simulink model "Exp5_MODEL_DCDC"  (R2023b)
settings: Solver=ode3  StartTime=0.0  StopTime=Time(end)  FixedStep=1e-6  RelTol=1e-3
undefined symbols (not defined in the file): C, L, LT1D_R_LOAD_1B, LT1D_R_LOAD_2B, R_L, R_lo_C, R_lo_nC_1B, R_lo_nC_2B, U_D, U_out
settings Model: Creator=tunkarlu  LastModifiedBy=tunkarlu

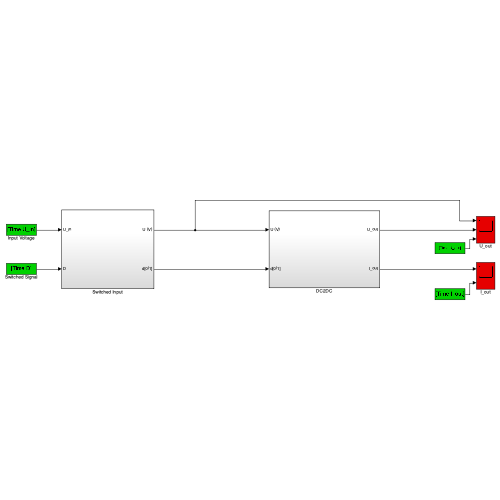
[thumbnail: Simulink's stored preview of the top-level diagram]
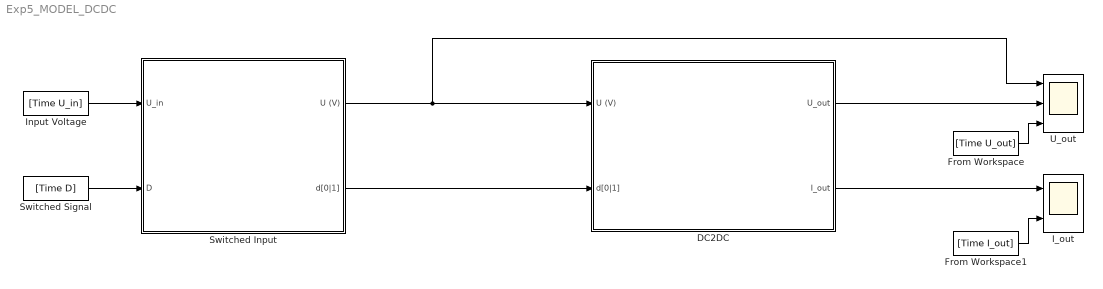
== system Exp5_MODEL_DCDC ==
  DC2DC : Subsystem
  From Workspace : FromWorkspace  VariableName=[Time U_out]
  From Workspace1 : FromWorkspace  VariableName=[Time I_out]
  I_out : Scope  NumInputPorts=2
  Input Voltage : FromWorkspace  VariableName=[Time U_in]
  Switched Input : Subsystem
  Switched Signal : FromWorkspace  VariableName=[Time D]
  U_out : Scope  NumInputPorts=3
  wires:
  Switched Signal/1 -> Switched Input/2(D)
  Input Voltage/1 -> Switched Input/1(U_in)
  From Workspace/1 -> U_out/3
  From Workspace1/1 -> I_out/2
  Switched Input/1(U (V)) -> U_out/1, DC2DC/1(U (V))
  Switched Input/2(d[0|1]) -> DC2DC/2(d[0|1])
  DC2DC/2(I_out) -> I_out/1
  DC2DC/1(U_out) -> U_out/2

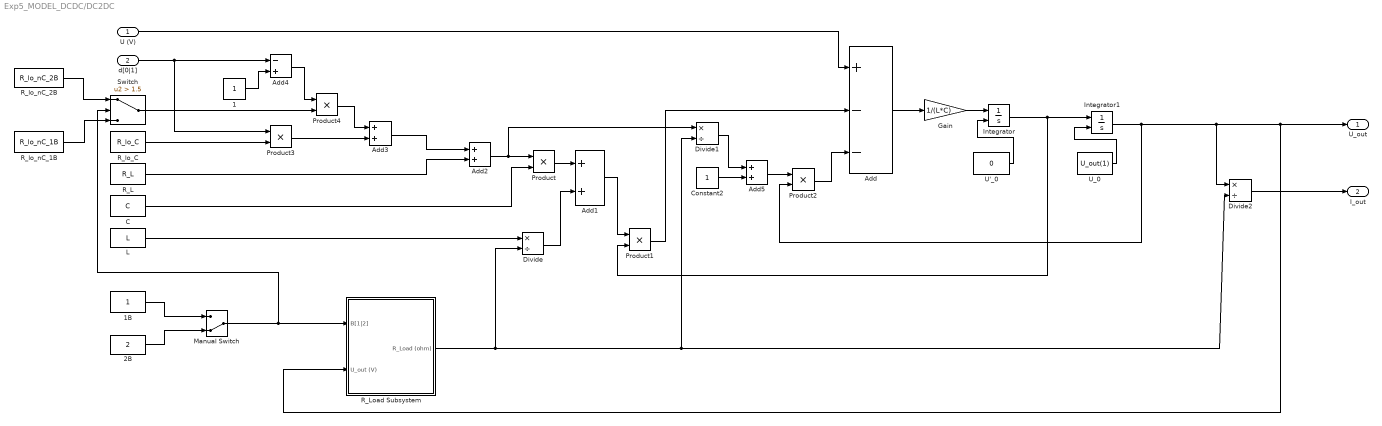
== system Exp5_MODEL_DCDC/DC2DC ==
  U (V) : Inport
  d[0|1] : Inport  Port=2
  1 : Constant
  1B : Constant
  2B : Constant  Value=2
  Add : Sum  Inputs=+--
  Add{1..3,5} (4 alike) : Sum
  Add4 : Sum  Inputs=-+
  C : Constant  Value=C
  Constant2 : Constant
  Divide : Product  Inputs=*/
  Divide1 : Product  Inputs=*/
  Divide2 : Product  Inputs=*/
  Gain : Gain  Gain=1/(L*C)
  Integrator : Integrator  InitialConditionSource=external
  Integrator1 : Integrator  InitialConditionSource=external
  L : Constant  Value=L
  Manual Switch : ManualSwitch  CurrentSetting=0
  Product{,1..4} (5 alike) : Product
  R_L : Constant  Value=R_L
  R_Load Subsystem : Subsystem
  R_lo_C : Constant  Value=R_lo_C
  R_lo_nC_1B : Constant  Value=R_lo_nC_1B
  R_lo_nC_2B : Constant  Value=R_lo_nC_2B
  Switch : Switch  Criteria=u2 > Threshold  Threshold=1.5  SaturateOnIntegerOverflow=off  InputSameDT=off
  U'_0 : Constant  Value=0
  U_0 : Constant  Value=U_out(1)
  U_out : Outport
  I_out : Outport  Port=2
  wires:
  R_L/1 -> Add2/2
  Divide1/1 -> Add5/1
  Add1/1 -> Product1/1
  1B/1 -> Manual Switch/1
  Manual Switch/1 -> Switch/2, R_Load Subsystem/1(B[1|2])
  Divide/1 -> Add1/2
  Product/1 -> Add1/1
  Product2/1 -> Add/3
  Integrator/1 -> Integrator1/1, Product1/2
  Divide2/1 -> I_out/1
  2B/1 -> Manual Switch/2
  R_Load Subsystem/1(R_Load (ohm)) -> Divide2/2, Divide1/2, Divide/2
  Product1/1 -> Add/2
  C/1 -> Product/2
  L/1 -> Divide/1
  Add/1 -> Gain/1
  Gain/1 -> Integrator/1
  Add2/1 -> Product/1, Divide1/1
  U (V)/1 -> Add/1
  Add3/1 -> Add2/1
  Integrator1/1 -> Divide2/1, U_out/1, R_Load Subsystem/2(U_out (V)), Product2/2
  R_lo_C/1 -> Product3/2
  d[0|1]/1 -> Product3/1, Add4/1
  1/1 -> Add4/2
  Add4/1 -> Product4/1
  Product4/1 -> Add3/1
  Product3/1 -> Add3/2
  U_0/1 -> Integrator1/2
  U'_0/1 -> Integrator/2
  Constant2/1 -> Add5/2
  Add5/1 -> Product2/1
  Switch/1 -> Product4/2
  R_lo_nC_1B/1 -> Switch/3
  R_lo_nC_2B/1 -> Switch/1

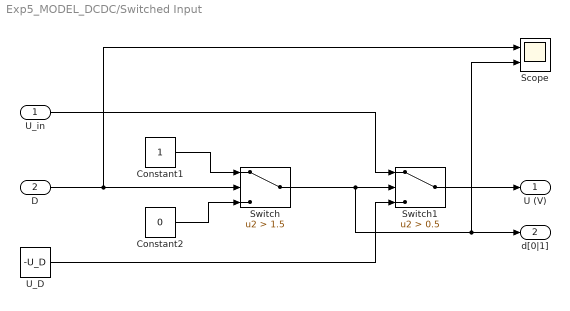
== system Exp5_MODEL_DCDC/Switched Input ==
  U_in : Inport
  D : Inport  Port=2
  Constant1 : Constant
  Constant2 : Constant  Value=0
  Scope : Scope  NumInputPorts=2
  Switch : Switch  Criteria=u2 > Threshold  Threshold=1.5  SaturateOnIntegerOverflow=off  InputSameDT=off
  Switch1 : Switch  Criteria=u2 > Threshold  Threshold=0.5  SaturateOnIntegerOverflow=off  InputSameDT=off
  U_D : Constant  Value=-U_D
  U (V) : Outport
  d[0|1] : Outport  Port=2
  wires:
  Switch1/1 -> U (V)/1
  Constant2/1 -> Switch/3
  D/1 -> Scope/1, Switch/2
  Constant1/1 -> Switch/1
  U_in/1 -> Switch1/1
  U_D/1 -> Switch1/3
  Switch/1 -> Switch1/2, Scope/2, d[0|1]/1

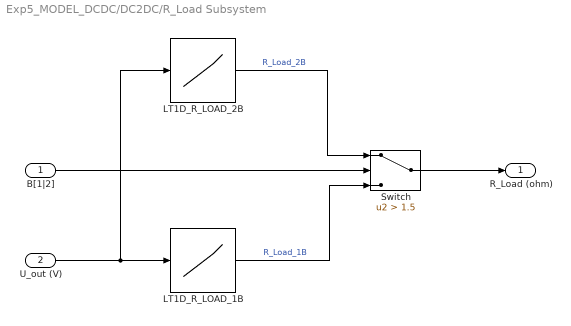
== system Exp5_MODEL_DCDC/DC2DC/R_Load Subsystem ==
  B[1|2] : Inport
  U_out (V) : Inport  Port=2
  LT1D_R_LOAD_1B : Lookup_n-D  NumberOfTableDimensions=1  BreakpointsForDimension1=LT1D_R_LOAD_1B(1,:)  Table=LT1D_R_LOAD_1B(2,:)  InternalRulePriority=Speed  RndMeth=Simplest
  LT1D_R_LOAD_2B : Lookup_n-D  NumberOfTableDimensions=1  BreakpointsForDimension1=LT1D_R_LOAD_2B(1,:)  Table=LT1D_R_LOAD_2B(2,:)  InternalRulePriority=Speed  RndMeth=Simplest
  Switch : Switch  Criteria=u2 > Threshold  Threshold=1.5  SaturateOnIntegerOverflow=off  InputSameDT=off
  R_Load (ohm) : Outport
  wires:
  B[1|2]/1 -> Switch/2
  Switch/1 -> R_Load (ohm)/1
  U_out (V)/1 -> LT1D_R_LOAD_2B/1, LT1D_R_LOAD_1B/1
  LT1D_R_LOAD_1B/1 -> Switch/3  "R_Load_1B"
  LT1D_R_LOAD_2B/1 -> Switch/1  "R_Load_2B"
